simulink model "Control_Block_a"  (R2020a)
settings: Solver=VariableStepAuto  StartTime=0.0  StopTime=10.0  RelTol=1e-3
libraries: fuzblock x6
settings Model: Creator=chris  LastModifiedBy=chris

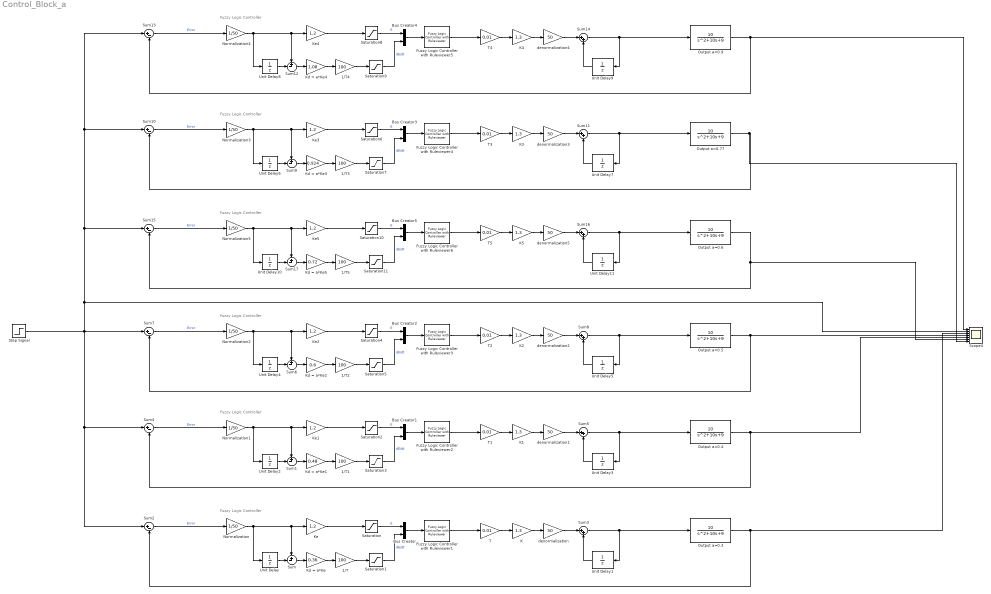
== system Control_Block_a ==
  note: Fuzzy Logic Controller
  note: Fuzzy Logic Controller
  note: Fuzzy Logic Controller
  note: Fuzzy Logic Controller
  note: Fuzzy Logic Controller
  note: Fuzzy Logic Controller
  1/T{,1..5} (6 alike) : Gain  Gain=100
  Bus Creator{,1..5} (6 alike) : BusCreator  Inputs=2
  Fuzzy Logic Controller with Ruleviewer{1..6} (6 alike) : fuzblock/Fuzzy Logic  Controller  with Ruleviewer  fismatrix=FLC  Ts=0.01
  K{,1..5} (6 alike) : Gain  Gain=1.3
  Kd = a*Ke : Gain  Gain=0.36
  Kd = a*Ke1 : Gain  Gain=0.48
  Kd = a*Ke2 : Gain  Gain=0.6
  Kd = a*Ke3 : Gain  Gain=0.924
  Kd = a*Ke4 : Gain  Gain=1.08
  Kd = a*Ke5 : Gain  Gain=0.72
  Ke{,1..5} (6 alike) : Gain  Gain=1.2
  Normalization{,1..5} (6 alike) : Gain  Gain=1/50
  Output a=0.{3..6,9,77} (6 alike) : TransferFcn  Numerator=[10]  Denominator=[1 10 9]
  Saturation{,1..11} (12 alike) : Saturate  UpperLimit=1  LowerLimit=-1
  Scope4 : Scope  NumInputPorts=7
  Step Signal : Step  Time=0  After=50  SampleTime=0.01
  Sum{,1,6,9,12,17} (6 alike) : Sum  Inputs=+-|
  Sum{2,4,7,10,13,15} (6 alike) : Sum  Inputs=|+-
  Sum{3,5,8,11,14,16} (6 alike) : Sum  Inputs=|++
  T{,1..5} (6 alike) : Gain  Gain=0.01
  Unit Delay{,1..11} (12 alike) : UnitDelay  SampleTime=-1  HasFrameUpgradeWarning=on
  denormalization{,1..5} (6 alike) : Gain  Gain=50
  wires:
  Step Signal/1 -> Sum7/1, Sum15/1, Sum13/1, Sum10/1, Scope4/2, Sum4/1, Sum2/1
  T4/1 -> K4/1
  Fuzzy Logic Controller with Ruleviewer5/1 -> T4/1
  denormalization4/1 -> Sum14/1
  Sum13/1 -> Normalization4/1  "Error"
  Kd = a*Ke4/1 -> 1/T4/1
  Bus Creator4/1 -> Fuzzy Logic Controller with Ruleviewer5/1
  Unit Delay8/1 -> Sum12/2
  Saturation8/1 -> Bus Creator4/1  "E"
  Sum12/1 -> Kd = a*Ke4/1
  Normalization4/1 -> Unit Delay8/1, Sum12/1, Ke4/1
  Output a=0.9/1 -> Scope4/1, Sum13/2
  Unit Delay9/1 -> Sum14/2
  Saturation9/1 -> Bus Creator4/2  "dE/dt"
  1/T4/1 -> Saturation9/1
  K4/1 -> denormalization4/1
  Ke4/1 -> Saturation8/1
  Sum14/1 -> Output a=0.9/1, Unit Delay9/1
  T3/1 -> K3/1
  Fuzzy Logic Controller with Ruleviewer4/1 -> T3/1
  denormalization3/1 -> Sum11/1
  Sum10/1 -> Normalization3/1  "Error"
  Kd = a*Ke3/1 -> 1/T3/1
  Bus Creator3/1 -> Fuzzy Logic Controller with Ruleviewer4/1
  Unit Delay6/1 -> Sum9/2
  Saturation6/1 -> Bus Creator3/1  "E"
  Sum9/1 -> Kd = a*Ke3/1
  Normalization3/1 -> Unit Delay6/1, Sum9/1, Ke3/1
  Output a=0.77/1 -> Scope4/7, Sum10/2
  Unit Delay7/1 -> Sum11/2
  Saturation7/1 -> Bus Creator3/2  "dE/dt"
  1/T3/1 -> Saturation7/1
  K3/1 -> denormalization3/1
  Ke3/1 -> Saturation6/1
  Sum11/1 -> Output a=0.77/1, Unit Delay7/1
  T2/1 -> K2/1
  Fuzzy Logic Controller with Ruleviewer3/1 -> T2/1
  denormalization2/1 -> Sum8/1
  Sum7/1 -> Normalization2/1  "Error"
  Kd = a*Ke2/1 -> 1/T2/1
  Bus Creator2/1 -> Fuzzy Logic Controller with Ruleviewer3/1
  Unit Delay4/1 -> Sum6/2
  Saturation4/1 -> Bus Creator2/1  "E"
  Sum6/1 -> Kd = a*Ke2/1
  Normalization2/1 -> Unit Delay4/1, Sum6/1, Ke2/1
  Output a=0.5/1 -> Scope4/4, Sum7/2
  Unit Delay5/1 -> Sum8/2
  Saturation5/1 -> Bus Creator2/2  "dE/dt"
  1/T2/1 -> Saturation5/1
  K2/1 -> denormalization2/1
  Ke2/1 -> Saturation4/1
  Sum8/1 -> Output a=0.5/1, Unit Delay5/1
  T1/1 -> K1/1
  Fuzzy Logic Controller with Ruleviewer2/1 -> T1/1
  denormalization1/1 -> Sum5/1
  Sum4/1 -> Normalization1/1  "Error"
  Kd = a*Ke1/1 -> 1/T1/1
  Bus Creator1/1 -> Fuzzy Logic Controller with Ruleviewer2/1
  Unit Delay2/1 -> Sum1/2
  Saturation2/1 -> Bus Creator1/1  "E"
  Sum1/1 -> Kd = a*Ke1/1
  Normalization1/1 -> Unit Delay2/1, Sum1/1, Ke1/1
  Output a=0.4/1 -> Sum4/2, Scope4/5
  Unit Delay3/1 -> Sum5/2
  Saturation3/1 -> Bus Creator1/2  "dE/dt"
  1/T1/1 -> Saturation3/1
  K1/1 -> denormalization1/1
  Ke1/1 -> Saturation2/1
  Sum5/1 -> Output a=0.4/1, Unit Delay3/1
  Sum2/1 -> Normalization/1  "Error"
  Sum3/1 -> Output a=0.3/1, Unit Delay1/1
  Output a=0.3/1 -> Sum2/2, Scope4/3
  1/T/1 -> Saturation1/1
  K/1 -> denormalization/1
  Unit Delay1/1 -> Sum3/2
  Saturation/1 -> Bus Creator/1  "E"
  Sum/1 -> Kd = a*Ke/1
  Unit Delay/1 -> Sum/2
  denormalization/1 -> Sum3/1
  Kd = a*Ke/1 -> 1/T/1
  Saturation1/1 -> Bus Creator/2  "dE/dt"
  T/1 -> K/1
  Ke/1 -> Saturation/1
  Normalization/1 -> Unit Delay/1, Sum/1, Ke/1
  Fuzzy Logic Controller with Ruleviewer1/1 -> T/1
  Bus Creator/1 -> Fuzzy Logic Controller with Ruleviewer1/1
  Kd = a*Ke5/1 -> 1/T5/1
  denormalization5/1 -> Sum16/1
  Output a=0.6/1 -> Scope4/6, Sum15/2
  Bus Creator5/1 -> Fuzzy Logic Controller with Ruleviewer6/1
  Saturation11/1 -> Bus Creator5/2  "dE/dt"
  1/T5/1 -> Saturation11/1
  Ke5/1 -> Saturation10/1
  K5/1 -> denormalization5/1
  Unit Delay10/1 -> Sum17/2
  Fuzzy Logic Controller with Ruleviewer6/1 -> T5/1
  T5/1 -> K5/1
  Saturation10/1 -> Bus Creator5/1  "E"
  Sum15/1 -> Normalization5/1  "Error"
  Sum17/1 -> Kd = a*Ke5/1
  Unit Delay11/1 -> Sum16/2
  Sum16/1 -> Output a=0.6/1, Unit Delay11/1
  Normalization5/1 -> Unit Delay10/1, Sum17/1, Ke5/1
